simulink model "mmcs_s2f"  (R2021b)
settings: Solver=FixedStepDiscrete  StartTime=0.0  StopTime=5  FixedStep=T_HF_TASK  RelTol=1e-3  EnableMultiTasking=on
PostLoadFcn:
  | run('init.m')
values from neighbouring files (symbols this model uses):
  ALIGN_DURATION = 700.0    [mmcs_s2f_dd.sldd]
  ALIGN_FINAL_CURRENT = 3277.0    [mmcs_s2f_dd.sldd]
  ALIGN_FINAL_SPEED = 0.0    [mmcs_s2f_dd.sldd]
  ALIGN_INIT_CURRENT = 1638.0    [mmcs_s2f_dd.sldd]
  ALIGN_THETA = 2731.0    [mmcs_s2f_dd.sldd]
  AMPTOS16 = 3277.0    [mmcs_s2f_dd.sldd]
  DIVSQRT_3 = 18918.0    [mmcs_s2f_dd.sldd]
  ENC_PT_CTRL = 4.0    [mmcs_s2f_dd.sldd]
  ENC_PULSE_NUM = 4000    [mmcs_s2f_dd.sldd]
  ENC_ST_CTRL = 2.0    [mmcs_s2f_dd.sldd]
  IF_ACC_DURATION = 1500.0    [mmcs_s2f_dd.sldd]
  IF_FINAL_CURRENT = 3277.0    [mmcs_s2f_dd.sldd]
  IF_FINAL_CURRENT_LOL = -3277.0    [mmcs_s2f_dd.sldd]
  IF_FINAL_CURRENT_UPL = 3277.0    [mmcs_s2f_dd.sldd]
  IF_FINAL_SPEED = 600.0    [mmcs_s2f_dd.sldd]
  IF_FINAL_SPEED_LOL = -600.0    [mmcs_s2f_dd.sldd]
  IF_FINAL_SPEED_UPL = 600.0    [mmcs_s2f_dd.sldd]
  IF_INIT_CURRENT = 1638.0    [mmcs_s2f_dd.sldd]
  INT16_MAX = 32767.0    [mmcs_s2f_dd.sldd]
  INT16_MIN = -32768.0    [mmcs_s2f_dd.sldd]
  MOTOR_F = 7.0E-6    [mmcs_s2f_dd.sldd]
  MOTOR_J = 2.8E-6    [mmcs_s2f_dd.sldd]
  MOTOR_PN = 4    [mmcs_s2f_dd.sldd]
  MOTOR_PNF = 4.0    [mmcs_s2f_dd.sldd]
  MOTOR_TL = 0.001    [mmcs_s2f_dd.sldd]
  PI_KI_PLL : value not decoded    [mmcs_s2f_dd.sldd]
  PI_KI_POS : value not decoded    [mmcs_s2f_dd.sldd]
  PI_KI_SPD : value not decoded    [mmcs_s2f_dd.sldd]
  PI_KI_TQ : value not decoded    [mmcs_s2f_dd.sldd]
  PI_KP_PLL : value not decoded    [mmcs_s2f_dd.sldd]
  PI_KP_POS : value not decoded    [mmcs_s2f_dd.sldd]
  PI_KP_SPD : value not decoded    [mmcs_s2f_dd.sldd]
  PI_KP_TQ : value not decoded    [mmcs_s2f_dd.sldd]
  PWM_FREQUENCY = 10000.0    [mmcs_s2f_dd.sldd]
  PWM_PERIOD_CYCLES = 7200.0    [mmcs_s2f_dd.sldd]
  RAD2RPM_F_DEN = 1000.0    [mmcs_s2f_dd.sldd]
  RAD2RPM_F_NUM = 9549.0    [mmcs_s2f_dd.sldd]
  RADTOS16_F = 10430.378350470453    [mmcs_s2f_dd.sldd]
  RADTOS16_I = 10430.0    [mmcs_s2f_dd.sldd]
  REF_CURRENT_LOL = -11470.0    [mmcs_s2f_dd.sldd]
  REF_CURRENT_UPL = 11470.0    [mmcs_s2f_dd.sldd]
  STM_ALIGN = 4.0    [mmcs_s2f_dd.sldd]
  STM_IFRUN = 5.0    [mmcs_s2f_dd.sldd]
  STM_INIT = 1.0    [mmcs_s2f_dd.sldd]
  STM_PTRUN = 7.0    [mmcs_s2f_dd.sldd]
  STM_START = 12.0    [mmcs_s2f_dd.sldd]
  STM_STRUN = 6.0    [mmcs_s2f_dd.sldd]
  STM_SWITCH = 11.0    [mmcs_s2f_dd.sldd]
  STO_C1 = 588    [mmcs_s2f_dd.sldd]
  STO_C2 = -5703    [mmcs_s2f_dd.sldd]
  STO_C3 = 1554    [mmcs_s2f_dd.sldd]
  STO_C4 = 7484    [mmcs_s2f_dd.sldd]
  STO_C5 = 1831    [mmcs_s2f_dd.sldd]
  STO_EST_MAX = 134213632.0    [mmcs_s2f_dd.sldd]
  STO_EST_MIN = -134213632.0    [mmcs_s2f_dd.sldd]
  STO_F1 = 4096.0    [mmcs_s2f_dd.sldd]
  STO_F2 = 4096.0    [mmcs_s2f_dd.sldd]
  STO_ST_CTRL = 3.0    [mmcs_s2f_dd.sldd]
  STOMS = 1000.0    [mmcs_s2f_dd.sldd]
  T_HF_TASK = 0.0001    [mmcs_s2f_dd.sldd]
  T_MF_TASK = 0.002    [mmcs_s2f_dd.sldd]
  TORQ_CTRL = 0.0    [mmcs_s2f_dd.sldd]
  U32MAXdivPulseNumber = 1073741    [mmcs_s2f_dd.sldd]
  VBUS = 24.0    [mmcs_s2f_dd.sldd]
undefined symbols (not defined in the file or in its folder): DiscIntNeverNeededParam
libraries: simulink x22, slpidlib x5, mcbplantlib x1, autolibpmsmexterior x1
(part 3 of 5)

== system mmcs_s2f/MFTask/SysCtrlModeUpdDet ==
  note: switch ENC_PT_CTRL
  sys_ctrl_mode : Inport  OutDataTypeStr=uint8
  pos_fed : Inport  Port=2  OutDataTypeStr=int32
  state : Inport  Port=3  OutDataTypeStr=uint8
  Compare To Constant : simulink/Logic and Bit Operations/Compare To Constant  relop===  const=ENC_PT_CTRL  OutDataTypeStr=boolean
  Compare To Constant1 : simulink/Logic and Bit Operations/Compare To Constant  relop===  const=ENC_ST_CTRL  OutDataTypeStr=boolean
  Compare To Constant4 : simulink/Logic and Bit Operations/Compare To Constant  relop===  const=STM_START  OutDataTypeStr=boolean
  Compare To Constant5 : simulink/Logic and Bit Operations/Compare To Constant  relop=~=  const=STM_START  OutDataTypeStr=boolean
  Compare To Constant6 : simulink/Logic and Bit Operations/Compare To Constant  relop===  const=ENC_PT_CTRL  OutDataTypeStr=boolean
  If : If  IfExpression=u1  ShowElse=off
  If Action Subsystem : Subsystem  TreatAsAtomicUnit=on
  Logical Operator : Logic  AllPortsSameDT=off  OutDataTypeStr=boolean
  Logical Operator2 : Logic  Operator=OR  AllPortsSameDT=off  OutDataTypeStr=boolean
  Logical Operator3 : Logic  Inputs=3  AllPortsSameDT=off  OutDataTypeStr=boolean
  Unit Delay : UnitDelay  SampleTime=-1  HasFrameUpgradeWarning=on
  Unit Delay1 : UnitDelay  SampleTime=-1  HasFrameUpgradeWarning=on
  wires:
  sys_ctrl_mode/1 -> Unit Delay/1, Compare To Constant6/1, Compare To Constant/1
  Logical Operator/1 -> Logical Operator2/1
  If/1 -> If Action Subsystem/Action
  Unit Delay/1 -> Compare To Constant1/1
  Compare To Constant/1 -> Logical Operator/1
  Compare To Constant1/1 -> Logical Operator/2
  pos_fed/1 -> If Action Subsystem/1(pos_fed)
  Logical Operator2/1 -> If/1
  state/1 -> Compare To Constant4/1, Unit Delay1/1
  Unit Delay1/1 -> Compare To Constant5/1
  Compare To Constant6/1 -> Logical Operator3/1
  Compare To Constant4/1 -> Logical Operator3/2
  Compare To Constant5/1 -> Logical Operator3/3
  Logical Operator3/1 -> Logical Operator2/2

== system mmcs_s2f/MFTask/TorqCtrl ==
  stm_state : Inport
  sys_ctrl_mode : Inport  Port=2  OutDataTypeStr=uint8
  spd_ref : Inport  Port=3  OutDataTypeStr=int16
  Action Port : ActionPort  ActionPortLabel=case [ 0 ]:
  AlignRamp : Subsystem
  AligntAction : Subsystem  TreatAsAtomicUnit=on
  Compare To Constant : simulink/Logic and Bit Operations/Compare To Constant  relop===  const=STM_START  OutDataTypeStr=uint8
  DefAction : Subsystem  TreatAsAtomicUnit=on
  IFRamp : Subsystem
  IFStart : Subsystem  TreatAsAtomicUnit=on
  Merge : Merge  Inputs=3
  Merge1 : Merge  Inputs=3
  Merge2 : Merge  Inputs=3
  Switch Case : SwitchCase  CaseConditions={STM_ALIGN,STM_IFRUN}
  Terminator : Terminator
  id_ref : Outport  OutDataTypeStr=int16
  iq_ref : Outport  Port=2  OutDataTypeStr=int16
  spd_ramp : Outport  Port=3  OutDataTypeStr=int16
  wires:
  stm_state/1 -> Compare To Constant/1, Switch Case/1
  Switch Case/1 -> AligntAction/Action
  Switch Case/2 -> IFStart/Action
  DefAction/1(id_ref) -> Merge/1
  AligntAction/1(id_ref) -> Merge/2
  IFStart/1(id_ref) -> Merge/3
  DefAction/2(iq_ref) -> Merge1/1
  AligntAction/2(iq_ref) -> Merge1/2
  IFStart/2(iq_ref) -> Merge1/3
  DefAction/3(spd_ramp) -> Merge2/1
  AligntAction/3(spd_ramp) -> Merge2/2
  IFStart/3(spd_ramp) -> Merge2/3
  Merge/1 -> id_ref/1
  Merge1/1 -> iq_ref/1
  Merge2/1 -> spd_ramp/1
  Switch Case/3 -> DefAction/Action
  sys_ctrl_mode/1 -> Terminator/1
  Compare To Constant/1 -> AlignRamp/1(reset), IFRamp/1(reset)
  IFRamp/1(id_ref) -> IFStart/1(id_ref_i)
  IFRamp/2(iq_ref) -> IFStart/2(iq_ref_i)
  IFRamp/3(spd_ramp) -> IFStart/3(spd_ramp_i)
  AlignRamp/1(id_ref) -> AligntAction/1(id_ref_i)
  AlignRamp/2(iq_ref) -> AligntAction/2(iq_ref_i)
  AlignRamp/3(spd_ramp) -> AligntAction/3(spd_ramp_i)
  spd_ref/1 -> IFRamp/2(spd_ref)

== system mmcs_s2f/SpeedConvert/SpdConvSim ==
  spd_sim : Inport
  Gain : Gain  Gain=30/pi  OutDataTypeStr=int16  RndMeth=Zero
  spd_fed : Outport
  wires:
  spd_sim/1 -> Gain/1
  Gain/1 -> spd_fed/1

== system mmcs_s2f/SpeedConvert/SpdConvSto ==
  w_dot : Inport  OutDataTypeStr=int16
  Constant1 : Constant  Value=RAD2RPM_F_NUM  OutDataTypeStr=uint16
  Constant3 : Constant  Value=RAD2RPM_F_DEN  OutDataTypeStr=uint16
  Divide : Product  Inputs=*/  OutDataTypeStr=int16  RndMeth=Zero
  GetAvgVal : MATLAB Function  TreatAsAtomicUnit=on
  Product : Product  OutDataTypeStr=int32  RndMeth=Zero
  spd_fed : Outport  OutDataTypeStr=int16
  wires:
  Constant3/1 -> Divide/2
  w_dot/1 -> Product/1
  Constant1/1 -> Product/2
  Product/1 -> Divide/1
  Divide/1 -> GetAvgVal/1(in_data)
  GetAvgVal/1(avg) -> spd_fed/1

== system mmcs_s2f/HFTask/AngleCalc/VssCalcAngle ==
  note: IF theta
  note: Align theta
  stm_state : Inport  OutDataTypeStr=uint8
  spd_ramp : Inport  Port=2  OutDataTypeStr=int16
  sys_ctrl_mode : Inport  Port=3  OutDataTypeStr=uint8
  Compare To Constant1 : simulink/Logic and Bit Operations/Compare To Constant  relop===  const=ENC_PT_CTRL  OutDataTypeStr=uint8
  Compare To Constant2 : simulink/Logic and Bit Operations/Compare To Constant  relop===  const=STM_ALIGN  OutDataTypeStr=uint8
  Compare To Constant3 : simulink/Logic and Bit Operations/Compare To Constant  relop===  const=ENC_ST_CTRL  OutDataTypeStr=uint8
  Constant1 : Constant  Value=0  OutDataTypeStr=int16
  Constant3 : Constant  Value=ALIGN_THETA  OutDataTypeStr=int16
  Constant4 : Constant  Value=0  OutDataTypeStr=int16
  EncCalcAngle : Subsystem
      settings: RTWFcnNameOpts=Use subsystem name  RTWFileNameOpts=Use subsystem name
  Logical Operator : Logic  Operator=OR  AllPortsSameDT=off  OutDataTypeStr=boolean
  Switch1 : Switch  Criteria=u2 > Threshold  RndMeth=Zero
  Switch2 : Switch  Criteria=u2 > Threshold  RndMeth=Zero
  VssEncoder : Subsystem
      settings: RTWFcnNameOpts=Use subsystem name  RTWFileNameOpts=Use subsystem name
  theta_e : Outport
  wires:
  VssEncoder/1(enc_cnt) -> EncCalcAngle/1(cnt)
  spd_ramp/1 -> VssEncoder/1(spd_ref)
  EncCalcAngle/1(theta_e) -> Switch1/3
  Constant1/1 -> VssEncoder/2(theta_0)
  stm_state/1 -> Compare To Constant2/1
  Compare To Constant2/1 -> VssEncoder/3(reset), Switch1/2
  Switch1/1 -> theta_e/1
  Switch2/1 -> Switch1/1
  Compare To Constant1/1 -> Logical Operator/2
  Constant3/1 -> Switch2/1
  Constant4/1 -> Switch2/3
  Compare To Constant3/1 -> Logical Operator/1
  Logical Operator/1 -> Switch2/2
  sys_ctrl_mode/1 -> Compare To Constant1/1, Compare To Constant3/1

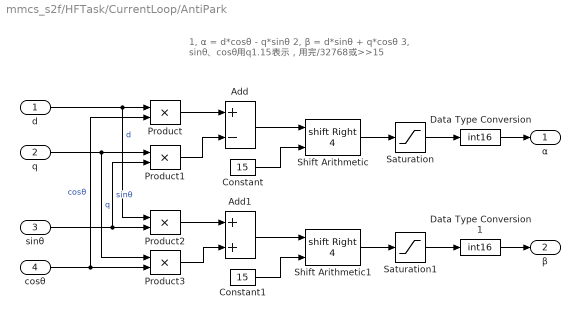
== system mmcs_s2f/HFTask/CurrentLoop/AntiPark ==
  note: 1, α = d*cosθ - q*sinθ
      | 2, β = d*sinθ + q*cosθ
      | 3, sinθ、cosθ用q1.15表示，用完/32768或>>15
  d : Inport  OutDataTypeStr=int16
  q : Inport  Port=2  OutDataTypeStr=int16
  sinθ : Inport  Port=3  OutDataTypeStr=int16
  cosθ : Inport  Port=4  OutDataTypeStr=int16
  Add : Sum  Inputs=+-  RndMeth=Zero
  Add1 : Sum  RndMeth=Zero
  Constant : Constant  Value=15  OutDataTypeStr=uint8
  Constant1 : Constant  Value=15  OutDataTypeStr=uint8
  Data Type Conversion : DataTypeConversion  OutDataTypeStr=int16  RndMeth=Zero
  Data Type Conversion1 : DataTypeConversion  OutDataTypeStr=int16  RndMeth=Zero
  Product{,1..3} (4 alike) : Product  RndMeth=Zero
  Saturation : Saturate  UpperLimit=INT16_MAX  LowerLimit=INT16_MIN  RndMeth=Zero
  Saturation1 : Saturate  UpperLimit=INT16_MAX  LowerLimit=INT16_MIN  RndMeth=Zero
  Shift Arithmetic : ArithShift  BitShiftNumberSource=Input port  BitShiftNumber=4  BitShiftDirection=Right
      settings: InputPortMap=u0,p1
  Shift Arithmetic1 : ArithShift  BitShiftNumberSource=Input port  BitShiftNumber=4  BitShiftDirection=Right
      settings: InputPortMap=u0,p1
  α : Outport
  β : Outport  Port=2
  wires:
  d/1 -> Product2/1, Product/1  "d"
  Add/1 -> Shift Arithmetic/1
  cosθ/1 -> Product/2, Product3/2  "cosθ"
  Constant/1 -> Shift Arithmetic/2
  Product1/1 -> Add/2
  q/1 -> Product3/1, Product1/1  "q"
  Product/1 -> Add/1
  sinθ/1 -> Product1/2, Product2/2  "sinθ"
  Add1/1 -> Shift Arithmetic1/1
  Data Type Conversion/1 -> α/1
  Constant1/1 -> Shift Arithmetic1/2
  Data Type Conversion1/1 -> β/1
  Product3/1 -> Add1/2
  Product2/1 -> Add1/1
  Shift Arithmetic/1 -> Saturation/1
  Saturation/1 -> Data Type Conversion/1
  Shift Arithmetic1/1 -> Saturation1/1
  Saturation1/1 -> Data Type Conversion1/1

== system mmcs_s2f/HFTask/CurrentLoop/Clark ==
  note: 1, i_alpha = ia
      | 2, i_beta = sqrt(3)/3 * (ia + 2*ib)
      | 3, sqrt(3)/3 = 0.57735; q1.15表示: 0.57735*32768 = 18918
      | 4, q1.15转int32: /32768或 >>15
  ia : Inport  OutDataTypeStr=int16
  ib : Inport  Port=2  OutDataTypeStr=int16
  Add : Sum  Inputs=+++  OutDataTypeStr=int32  RndMeth=Zero
  Constant : Constant  Value=15  OutDataTypeStr=uint8
  Data Type Conversion : DataTypeConversion  OutDataTypeStr=int16  RndMeth=Zero
  Data Type Conversion1 : DataTypeConversion  OutDataTypeStr=int16  RndMeth=Zero
  Gain4 : Gain  Gain=DIVSQRT_3  OutDataTypeStr=int32  RndMeth=Zero
  Saturation : Saturate  UpperLimit=INT16_MAX  LowerLimit=INT16_MIN  RndMeth=Zero
  Shift Arithmetic : ArithShift  BitShiftNumberSource=Input port  BitShiftNumber=4  BitShiftDirection=Right
      settings: InputPortMap=u0,p1
  i_alpha : Outport  OutDataTypeStr=int16
  i_beta : Outport  Port=2  OutDataTypeStr=int16
  wires:
  Gain4/1 -> Shift Arithmetic/1
  ib/1 -> Add/3, Add/2
  Add/1 -> Gain4/1
  Constant/1 -> Shift Arithmetic/2
  Shift Arithmetic/1 -> Saturation/1
  Saturation/1 -> Data Type Conversion/1
  ia/1 -> Data Type Conversion1/1, Add/1
  Data Type Conversion/1 -> i_beta/1
  Data Type Conversion1/1 -> i_alpha/1

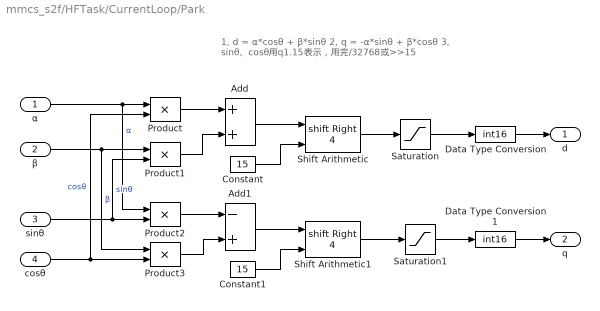
== system mmcs_s2f/HFTask/CurrentLoop/Park ==
  note: 1, d = α*cosθ + β*sinθ
      | 2, q = -α*sinθ + β*cosθ
      | 3, sinθ、cosθ用q1.15表示，用完/32768或>>15
  α : Inport  OutDataTypeStr=int16
  β : Inport  Port=2  OutDataTypeStr=int16
  sinθ : Inport  Port=3  OutDataTypeStr=int16
  cosθ : Inport  Port=4  OutDataTypeStr=int16
  Add : Sum  RndMeth=Zero
  Add1 : Sum  Inputs=-+  RndMeth=Zero
  Constant : Constant  Value=15  OutDataTypeStr=uint8
  Constant1 : Constant  Value=15  OutDataTypeStr=uint8
  Data Type Conversion : DataTypeConversion  OutDataTypeStr=int16  RndMeth=Zero
  Data Type Conversion1 : DataTypeConversion  OutDataTypeStr=int16  RndMeth=Zero
  Product{,1..3} (4 alike) : Product  RndMeth=Zero
  Saturation : Saturate  UpperLimit=INT16_MAX  LowerLimit=INT16_MIN  RndMeth=Zero
  Saturation1 : Saturate  UpperLimit=INT16_MAX  LowerLimit=INT16_MIN  RndMeth=Zero
  Shift Arithmetic : ArithShift  BitShiftNumberSource=Input port  BitShiftNumber=4  BitShiftDirection=Right
      settings: InputPortMap=u0,p1
  Shift Arithmetic1 : ArithShift  BitShiftNumberSource=Input port  BitShiftNumber=4  BitShiftDirection=Right
      settings: InputPortMap=u0,p1
  d : Outport
  q : Outport  Port=2
  wires:
  Add/1 -> Shift Arithmetic/1
  Shift Arithmetic/1 -> Saturation/1
  Constant/1 -> Shift Arithmetic/2
  α/1 -> Product2/1, Product/1  "α"
  cosθ/1 -> Product/2, Product3/2  "cosθ"
  β/1 -> Product3/1, Product1/1  "β"
  sinθ/1 -> Product1/2, Product2/2  "sinθ"
  Product/1 -> Add/1
  Product1/1 -> Add/2
  Product2/1 -> Add1/1
  Product3/1 -> Add1/2
  Constant1/1 -> Shift Arithmetic1/2
  Add1/1 -> Shift Arithmetic1/1
  Saturation/1 -> Data Type Conversion/1
  Shift Arithmetic1/1 -> Saturation1/1
  Saturation1/1 -> Data Type Conversion1/1
  Data Type Conversion/1 -> d/1
  Data Type Conversion1/1 -> q/1

== system mmcs_s2f/HFTask/CurrentLoop/Subsystem ==
  mode : Inport  OutDataTypeStr=uint8
  Compare To Constant : simulink/Logic and Bit Operations/Compare To Constant  relop=~=  const=ENC_PT_CTRL  OutDataTypeStr=uint8
  Constant : Constant  Value=PI_KP_TQ  OutDataTypeStr=fixdt(1,32,16)
  Constant1 : Constant  Value=PI_KI_TQ/15  OutDataTypeStr=fixdt(1,32,16)
  Constant2 : Constant  Value=PI_KI_TQ  OutDataTypeStr=fixdt(1,32,16)
  Switch : Switch  Criteria=u2 > Threshold
  KP : Outport
  KI : Outport  Port=2
  wires:
  mode/1 -> Compare To Constant/1
  Compare To Constant/1 -> Switch/2
  Constant1/1 -> Switch/3
  Constant2/1 -> Switch/1
  Constant/1 -> KP/1
  Switch/1 -> KI/1

== system mmcs_s2f/HFTask/ObserverPLL/Resettable Subsystem ==
  u_alpha_beta : Inport  OutDataTypeStr=int16
  i_alpha_beta : Inport  Port=2  OutDataTypeStr=int16
  reset : Inport  Port=3  OutDataTypeStr=uint8
  spd_ref : Inport  Port=4  OutDataTypeStr=int16
  Reset : ResetPort  DisableCoverage=on
  Constant : Constant  Value=MOTOR_PN
  Divide : Product  Inputs=*/  RndMeth=Zero
  Observer : Subsystem
      settings: RTWFcnNameOpts=Use subsystem name  RTWFileNameOpts=Use subsystem name
  PLL : Subsystem
      settings: RTWFcnNameOpts=Use subsystem name  RTWFileNameOpts=Use subsystem name
  Unit Delay8 : UnitDelay  SampleTime=-1  HasFrameUpgradeWarning=on
  theta_e_dot : Outport  OutDataTypeStr=int16
  w_dot : Outport  Port=2  OutDataTypeStr=int16
  iα_dot_next : Outport  Port=3  OutDataTypeStr=int32
  iβ_dot_next : Outport  Port=4  OutDataTypeStr=int32
  wires:
  spd_ref/1 -> PLL/4(spd_ref)
  reset/1 -> PLL/3(reset)
  Unit Delay8/1 -> Observer/3(we_dot)
  Observer/2(iβ_dot_next) -> iβ_dot_next/1  "i_beta_dot"
  u_alpha_beta/1 -> Observer/1(u_αβ)
  Observer/3(eα_dot_next) -> PLL/1(eα_dot)  "e_alpha_dot"
  i_alpha_beta/1 -> Observer/2(i_αβ)
  PLL/2(we_dot) -> Unit Delay8/1, Divide/1
  Divide/1 -> w_dot/1
  Observer/4(eβ_dot_next) -> PLL/2(eβ_dot)  "e_beta_dot"
  PLL/1(theta_e_dot) -> theta_e_dot/1
  Constant/1 -> Divide/2
  Observer/1(iα_dot_next) -> iα_dot_next/1  "i_alpha_dot"

== system mmcs_s2f/MFTask/IsTransition/If Action Subsystem ==
  spd_dot : Inport
  Action Port : ActionPort  ActionPortLabel=if(u1)
  Abs : Abs  RndMeth=Zero
  Constant1 : Constant  Value=IF_FINAL_SPEED
  Constant2 : Constant  Value=9  OutDataTypeStr=uint8
  Constant3 : Constant  Value=10  OutDataTypeStr=uint8
  Constant4 : Constant  Value=11  OutDataTypeStr=uint8
  Constant5 : Constant  Value=10  OutDataTypeStr=uint8
  Divide : Product  Inputs=*/  OutDataTypeStr=int16  RndMeth=Zero
  Divide1 : Product  Inputs=*/  OutDataTypeStr=int16  RndMeth=Zero
  Logical Operator : Logic  AllPortsSameDT=off  OutDataTypeStr=boolean
  Product : Product  OutDataTypeStr=int16  RndMeth=Zero
  Product1 : Product  OutDataTypeStr=int16  RndMeth=Zero
  Relational Operator : RelationalOperator  OutDataTypeStr=boolean  RndMeth=Zero
  Relational Operator1 : RelationalOperator  Operator=<=  OutDataTypeStr=boolean  RndMeth=Zero
  transition : Outport
  wires:
  Divide/1 -> Relational Operator/2
  spd_dot/1 -> Abs/1
  Divide1/1 -> Relational Operator1/2
  Relational Operator/1 -> Logical Operator/1
  Relational Operator1/1 -> Logical Operator/2
  Logical Operator/1 -> transition/1
  Product/1 -> Divide/1
  Constant2/1 -> Product/2
  Constant3/1 -> Divide/2
  Constant5/1 -> Divide1/2
  Constant4/1 -> Product1/2
  Product1/1 -> Divide1/1
  Constant1/1 -> Product1/1, Product/1
  Abs/1 -> Relational Operator1/1, Relational Operator/1

== system mmcs_s2f/MFTask/PosCtrl/If Action Subsystem ==
  pos_ctrl : Inport  OutDataTypeStr=Bus: PosCtrlHandle_t
  Action Port : ActionPort  ActionPortLabel=if(u1 > 0)
  Data Store Write : DataStoreWrite  DataStoreName=pos_ctrl  DataStoreElements=pos_ctrl  IndexOptions=Index vector (dialog)  Indices=1  OutputSizes=1
  wires:
  pos_ctrl/1 -> Data Store Write/1

== system mmcs_s2f/MFTask/PosCtrl/PosControler ==
  reset : Inport  OutDataTypeStr=uint8
  pos_ref : Inport  Port=2  OutDataTypeStr=int32
  pos_fed : Inport  Port=3  OutDataTypeStr=int32
  plan_exec : Inport  Port=4  OutDataTypeStr=uint8
  Constant6 : Constant  Value=0  OutDataTypeStr=int16
  Data Type Conversion : DataTypeConversion  OutDataTypeStr=int16  RndMeth=Zero
  PosControler : slpidlib/PID Controller  Controller=PI  Form=Parallel  TimeDomain=Discrete-time  UseExternalTs=off  SampleTime=-1  IntegratorMethod=Forward Euler  FilterMethod=Forward Euler  ControllerParametersSource=internal  P=PI_KP_POS  I=PI_KI_POS  D=0  UseFilter=on  N=100  TunerSelectOption=Transfer Function Based (PID Tuner App)  InitialConditionSource=internal  InitialConditionForIntegrator=0  InitialConditionForFilter=0  DifferentiatorICPrevScaledInput=0  ExternalReset=level  TrackingMode=off  Kt=1  LimitOutput=on  SatLimitsSource=internal  UpperSaturationLimit=INT16_MAX  LowerSaturationLimit=INT16_MIN  LinearizeAsGain=off  AntiWindupMode=clamping  Kb=1  RndMeth=Zero  POutMin=[]  POutMax=[]  IOutMin=[]  IOutMax=[]  DOutMin=[]  DOutMax=[]  NOutMin=[]  NOutMax=[]  SumOutDataTypeStr=int32  SumOutMin=[]  SumOutMax=[]  SaturationOutDataTypeStr=int32  SaturationOutMin=[]  SaturationOutMax=[]  PParamMin=[]  PParamMax=[]  IParamMin=[]  IParamMax=[]  DParamMin=[]  DParamMax=[]  NParamMin=[]  NParamMax=[]  KbParamMin=[]  KbParamMax=[]  KtParamMin=[]  KtParamMax=[]  KbOutMin=[]  KbOutMax=[]  KtOutMin=[]  KtOutMax=[]  IntegratorOutMin=[]  IntegratorOutMax=[]  FilterOutMin=[]  FilterOutMax=[]  SumI1OutMin=[]  SumI1OutMax=[]  SumI2OutMin=[]  SumI2OutMax=[]  SumI3OutMin=[]  SumI3OutMax=[]  SumI4OutMin=[]  SumI4OutMax=[]  SumDOutMin=[]  SumDOutMax=[]  DifferentiatorOutMin=[]  DifferentiatorOutMax=[]  FilterDiffOutCoefMin=[]  FilterDiffOutCoefMax=[]  ReciprocalOutMin=[]  ReciprocalOutMax=[]  SumDenOutMin=[]  SumDenOutMax=[]  SumNumOutMin=[]  SumNumOutMax=[]  DivideOutMin=[]  DivideOutMax=[]  UdiffTsProdOutMin=[]  UdiffTsProdOutMax=[]  NTsProdOutMin=[]  NTsProdOutMax=[]  UintegralTsProdOutMin=[]  UintegralTsProdOutMax=[]  UngainTsProdOutMin=[]  UngainTsProdOutMax=[]  IntegratorContinuousStateAttributes=''  IntegratorStateMustResolveToSignalObject=off  IntegratorRTWStateStorageClass=Auto  FilterContinuousStateAttributes=''  FilterStateMustResolveToSignalObject=off  FilterRTWStateStorageClass=Auto  ParallelPVariant=InternalParameters  IdealPVariant=Disabled  IVariant=InternalParameters  DVariant=Disabled  IntegratorVariant=Discrete  SatVariant=Enabled  AWVariant=DiscClampingParallel  PCopyVariant=Disabled  TRVariant=Disabled  FdbkBlocksVariant=Forward  IdealPFdbkVariant=Disabled  SatFdbkVariant=Disabled  DerivativeFilterVariant=Disabled  NVariant=Disabled  NCopyVariant=Disabled_SignalSpec  FilterICVariant=Disabled  IntegratorICVariant=InternalICs  ExternalResetVariant=ExternalReset  TRSumVariant=Passthrough  SumFdbkVariant=Disabled  SumVariant=Sum_PI  TsampFilterVariant=InternalTs  TsampNgainVariant=Passthrough  TsampIntegralVariant=Passthrough  ExternalSaturationOutDataTypeStr=Inherit: Same as second input
  Scope : Scope  NumInputPorts=2
  Sum : Sum  Inputs=|+-  RndMeth=Zero
  Terminator : Terminator
  id_ref : Outport  OutDataTypeStr=int16
  iq_ref : Outport  Port=2  OutDataTypeStr=int16
  wires:
  reset/1 -> PosControler/2
  Data Type Conversion/1 -> iq_ref/1
  PosControler/1 -> Data Type Conversion/1
  pos_fed/1 -> Scope/2, Sum/2
  pos_ref/1 -> Sum/1, Scope/1  "pos_ref_int"
  Sum/1 -> PosControler/1
  Constant6/1 -> id_ref/1
  plan_exec/1 -> Terminator/1

== system mmcs_s2f/MFTask/PosCtrlInit/PosCtrlInit ==
  Action Port : ActionPort  ActionPortLabel=if(u1)
  Data Store Write : DataStoreWrite  DataStoreName=pos_ctrl  DataStoreElements=pos_ctrl  IndexOptions=Index vector (dialog)  Indices=1  OutputSizes=1
  sfun_PosCtrlInit : S-Function  FunctionName=sfun_PosCtrlInit  SFunctionDeploymentMode=off  EnableBusSupport=off  mask(Legacy Function){SFunctionSpec=void PosCtrlInit(PosCtrlHandle_t y1[1]), ShowSpec=off}
      mask prompts: ShowSpec "显示函数设定"
      mask help:
      | 此模块允许您调用由以下代码继承工具定义指定的已有函数:
      | def.SFunctionName = 'sfun_PosCtrlInit';
      | def.OutputFcnSpec = 'void PosCtrlInit(PosCtrlHandle_t y1[1])';
      | def.HeaderFiles = {'trajectory_ctrl.h'};
      mask Help: <p>此模块是由代码继承工具自动生成的。有关此工具的详细帮助，请调用<a href="matlab:legacy_code('help')"> legacy_code('help')</a>.</p>
      mask Callback ShowSpec:
      | if strcmp(get_param(gcbh, 'ShowSpec'), 'on')
      |   set_param(gcbh, 'MaskDisplay', sprintf('fprintf(''%s'');', get_param(gcbh, 'SFunctionSpec')));
      | else
      |   set_param(gcbh, 'MaskDisplay', sprintf('fprintf(''%s'');', get_param(gcbh, 'FunctionName')));
      | end
      mask Display: fprintf('sfun_PosCtrlInit');
  wires:
  sfun_PosCtrlInit/1 -> Data Store Write/1

== system mmcs_s2f/MFTask/PosCtrlPlan/PosCtrlPlan ==
  pos_fed : Inport
  pos_ref : Inport  Port=2
  duration : Inport  Port=3
  Action Port : ActionPort  ActionPortLabel=if(u1)
  Constant2 : Constant  Value=RADTOS16_F  OutDataTypeStr=single
  Data Store Read : DataStoreRead  DataStoreName=pos_ctrl  DataStoreElements=pos_ctrl  IndexOptions=Index vector (dialog)  Indices=1  OutputSizes=1
  Divide : Product  Inputs=*/  OutDataTypeStr=single  RndMeth=Zero
  If : If  ShowElse=off
  UpdatePosCtrl : Subsystem  TreatAsAtomicUnit=on
  sfun_PosCtrPlan : S-Function  FunctionName=sfun_PosCtrPlan  SFunctionDeploymentMode=off  EnableBusSupport=off  mask(Legacy Function){SFunctionSpec=uint8 y1 = PosCtrPlan(single u1, single u2, single u3, PosCtrlHandle_t u4[1], PosCtrlHandle_t y2[1]), ShowSpec=off}
      mask prompts: ShowSpec "显示函数设定"
      mask help:
      | 此模块允许您调用由以下代码继承工具定义指定的已有函数:
      | def.SFunctionName = 'sfun_PosCtrPlan';
      | def.OutputFcnSpec = 'uint8 y1 = PosCtrPlan(single u1, single u2, single u3, PosCtrlHandle_t u4[1], PosCtrlHandle_t y2[1])';
      | def.HeaderFiles = {'trajectory_ctrl.h'};
      mask Help: <p>此模块是由代码继承工具自动生成的。有关此工具的详细帮助，请调用<a href="matlab:legacy_code('help')"> legacy_code('help')</a>.</p>
      mask Callback ShowSpec:
      | if strcmp(get_param(gcbh, 'ShowSpec'), 'on')
      |   set_param(gcbh, 'MaskDisplay', sprintf('fprintf(''%s'');', get_param(gcbh, 'SFunctionSpec')));
      | else
      |   set_param(gcbh, 'MaskDisplay', sprintf('fprintf(''%s'');', get_param(gcbh, 'FunctionName')));
      | end
      mask Display: fprintf('sfun_PosCtrPlan');
  wires:
  Constant2/1 -> Divide/2
  duration/1 -> sfun_PosCtrPlan/3
  pos_fed/1 -> Divide/1
  pos_ref/1 -> sfun_PosCtrPlan/2
  Divide/1 -> sfun_PosCtrPlan/1
  Data Store Read/1 -> sfun_PosCtrPlan/4
  sfun_PosCtrPlan/1 -> If/1
  If/1 -> UpdatePosCtrl/Action
  sfun_PosCtrPlan/2 -> UpdatePosCtrl/1(pos_ctrl)
